simulink model "simulateQPSK_pulseShapingRectangular_variableNoise"  (R2017a)
settings: Solver=VariableStepAuto  StartTime=0.0  StopTime=inf  RelTol=1e-3
InitFcn:
  | Tb = 1/1000;        % bit time
  | Tsym = Tb * 2;   % QPSK encodes 2 bits per symbol
  | frameSize = 1000;
libraries: commutil2 x2, commfilt2 x2, commdigbbndpm3 x2, commchan3 x1, commrandsrc3 x1, simulink x1
settings Model: Creator=prust  LastModifiedBy=prust

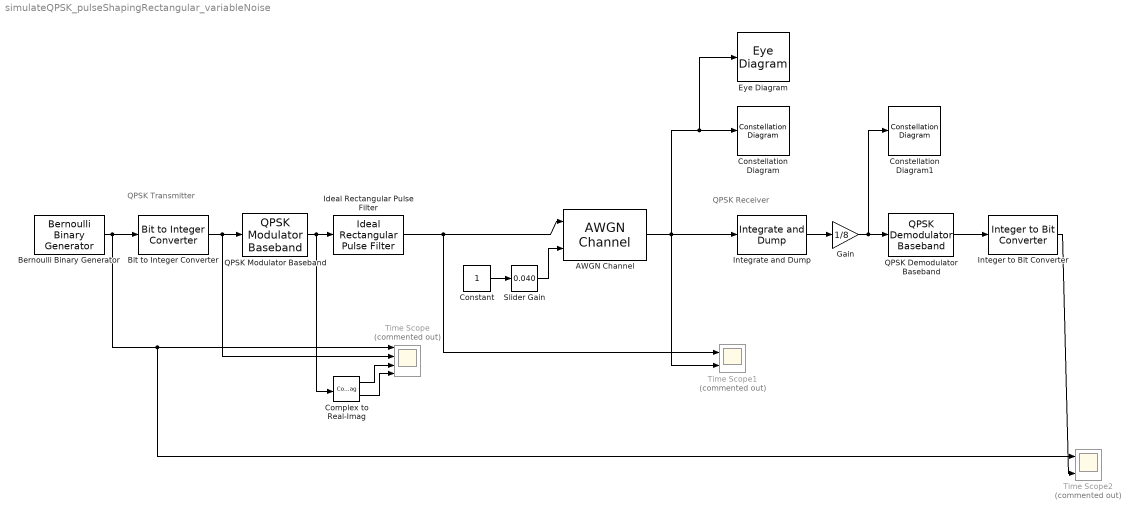
== system simulateQPSK_pulseShapingRectangular_variableNoise ==
  note: QPSK Receiver
  note: QPSK Transmitter
  AWGN Channel : commchan3/AWGN Channel  InputProcessing=Columns as channels (frame based)  seed=67  noiseMode=Variance from port  EbNodB=15  EsNodB=10  SNRdB=10  bitsPerSym=2  Ps=1  Tsym=Tsym  variance=1
  Bernoulli Binary Generator : commrandsrc3/Bernoulli Binary Generator  ProbabilityOfZero=0.5  SeedSource=Auto  Seed=0  SampleTime=Tb  SamplesPerFrame=frameSize  OutputDataType=double  SimulateUsing=Interpreted execution
  Bit to Integer Converter : commutil2/Bit to Integer Converter  nbits=2  bitOrder=MSB first  signedOutputValues=Unsigned  outDtype=Inherit via internal rule  outDtypeSigned=Inherit via internal rule
  Complex to Real-Imag : ComplexToRealImag
  Constant : Constant
  Constellation Diagram : ConstellationDiagram
  Constellation Diagram1 : ConstellationDiagram
  Eye Diagram : EyeDiagram
  Gain : Gain  Gain=1/8
  Ideal Rectangular Pulse Filter : commfilt2/Ideal Rectangular Pulse Filter  pulseLen=8  pulseDelay=0  InputProcessing=Columns as channels (frame based)  RateOptions=Enforce single-rate processing  sampMode=Mute  normCheck=off  normMode=Sum of samples  filterGain=1  saveAsFlag=0  roundingMode=Floor  overflowMode=off  firstCoeffDataTypeStr=Inherit: Same word length as input  firstCoeffMin=[]  firstCoeffMax=[]  firstCoeffLastDataTypeStr=Inherit: Same word length as input  outputDataTypeStr=Inherit: Same as accumulator  outputMin=[]  outputMax=[]  outputLastDataTypeStr=Inherit: Same as accumulator
      settings: SourceProductName=Communications System Toolbox  SourceProductBaseCode=CM
  Integer to Bit Converter : commutil2/Integer to Bit Converter  nbits=2  signedInputValues=Unsigned  bitOrder=MSB first  outDtype=Inherit via internal rule
  Integrate and Dump : commfilt2/Integrate and Dump  obssamples=8  offsetsamples=0  nodump=off  roundingMode=Floor  overflowMode=off  outputDataTypeStr=Inherit: Same as accumulator  outputLastDataTypeStr=Inherit: Same as accumulator
      settings: SourceProductName=Communications System Toolbox
  QPSK Demodulator Baseband : commdigbbndpm3/QPSK Demodulator Baseband  OutType=Integer  DecType=Hard decision  VarSource=Dialog  Variance=1  Dec=Gray  Ph=pi/4  outDtype1=Inherit via internal rule  outDtype2=Inherit via internal rule  derotateFactorWordLen=16  derotateFactorDataTypeStr=Inherit: Same word length as input  derotateFactorLastDataTypeStr=Inherit: Same word length as input
  QPSK Modulator Baseband : commdigbbndpm3/QPSK Modulator Baseband  InType=Integer  Enc=Gray  Ph=pi/4  outDtype=double  outWordLen=16  outUDDataType=sfix(16)  outFracLenMode=Best precision  outFracLen=15  outDataTypeStr=double  outLastDataTypeStr=double
  Slider Gain : simulink/Math Operations/Slider Gain  gain=0.040  low=0  high=2
  Time Scope : Scope  Commented=on  NumInputPorts=4
  Time Scope1 : Scope  Commented=on  NumInputPorts=2
  Time Scope2 : Scope  Commented=on  NumInputPorts=2
  wires:
  Bit to Integer Converter/1 -> Time Scope/2, QPSK Modulator Baseband/1
  QPSK Modulator Baseband/1 -> Ideal Rectangular Pulse Filter/1, Complex to Real-Imag/1
  AWGN Channel/1 -> Integrate and Dump/1, Time Scope1/2, Eye Diagram/1, Constellation Diagram/1
  QPSK Demodulator Baseband/1 -> Integer to Bit Converter/1
  Bernoulli Binary Generator/1 -> Time Scope2/1, Time Scope/1, Bit to Integer Converter/1
  Ideal Rectangular Pulse Filter/1 -> AWGN Channel/1, Time Scope1/1
  Gain/1 -> Constellation Diagram1/1, QPSK Demodulator Baseband/1
  Complex to Real-Imag/1 -> Time Scope/3
  Complex to Real-Imag/2 -> Time Scope/4
  Constant/1 -> Slider Gain/1
  Slider Gain/1 -> AWGN Channel/2
  Integrate and Dump/1 -> Gain/1
  Integer to Bit Converter/1 -> Time Scope2/2
